simulink model "Punto_8"  (R2020a)
settings: Solver=VariableStepAuto  StartTime=0.0  StopTime=10.0  RelTol=1e-3
undefined symbols (not defined in the file): A, B
settings Model: Creator=nicoquintero  LastModifiedBy=nicoquintero

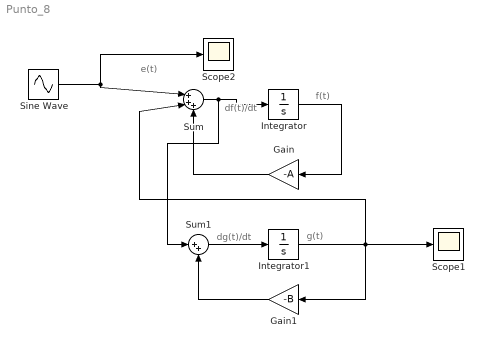
== system Punto_8 ==
  note: e(t)
  note: g(t)
  note: dg(t)/dt
  note: f(t)
  note: df(t)/dt
  Gain : Gain  Gain=-A
  Gain1 : Gain  Gain=-B
  Integrator : Integrator
  Integrator1 : Integrator
  Scope1 : Scope
  Scope2 : Scope
  Sine Wave : Sin  Frequency=B  Phase=pi/2+A  SampleTime=0
  Sum : Sum  Inputs=|+++
  Sum1 : Sum  Inputs=|++
  wires:
  Integrator/1 -> Gain/1
  Sum/1 -> Sum1/1, Integrator/1
  Integrator1/1 -> Sum/2, Scope1/1, Gain1/1
  Gain/1 -> Sum/3
  Gain1/1 -> Sum1/2
  Sum1/1 -> Integrator1/1
  Sine Wave/1 -> Sum/1, Scope2/1
